simulink model "DSB_SC_coherent_2020b"  (R2020b)
settings: Solver=ode45  StartTime=0.0  StopTime=50  RelTol=1e-3  EnableMultiTasking=on
values from neighbouring files (symbols this model uses):
  seed = input('Enter your student ID: ')    [DSBAMsignals.m]    (also in DSBAMsignals_rand.m; DSB_SC_sinusoidals.m)
libraries: dsparch4 x2
settings Model: Creator=morelos_zaragoza  LastModifiedBy=14083
settings DataIOCC: LimitDataPoints=on  SaveFormat=Array  SignalLoggingSaveFormat=ModelDataLogs  ReturnWorkspaceOutputs=off
settings OptimizationCC: ExpressionDepthLimit=2147483647  InitFltsAndDblsToZero=on  LifeSpan=inf
settings DebuggingCC: SaveWithParameterizedLinksMsg=none  UnderspecifiedInitializationDetection=Classic  MergeDetectMultiDrivingBlocksExec=none  SignalResolutionControl=TryResolveAllWithWarning  SolverPrmCheckMsg=warning  MultiTaskDSMMsg=warning  MultiTaskCondExecSysMsg=none  FcnCallInpInsideContextMsg=warning  StateNameClashWarn=warning  SFUnexpectedBacktrackingDiag=warning  SFNoUnconditionalDefaultTransitionDiag=warning  SFExecutionAtInitializationDiag=none  ArithmeticOperatorsInVariantConditions=warning
settings HardwareCC: ProdBitPerPointer=32  ProdBitPerSizeT=32  ProdBitPerPtrDiffT=32  ProdLargestAtomicFloat=None  ProdIntDivRoundTo=Undefined  ProdEndianess=Unspecified  ProdWordSize=32  ProdHWDeviceType=32-bit Generic
settings ModelReferenceCC: PropagateSignalLabelsOutOfModel=off
settings SFSimCC: SimUseLocalCustomCode=off  CustomCodeUndefinedFunction=UseInterfaceOnly
settings RTWCC: RTWUseLocalCustomCode=off
settings CodeAppCC: StateflowObjectComments=on
settings GRTTargetCC: TargetFcnLib=ansi_tfl_tmw.mat  TargetLangStandard=C89/C90 (ANSI)  CombineOutputUpdateFcns=off  GRTInterface=on
settings ConfigComp: CovMetricSettings=dw  CovSaveCumulativeToWorkspaceVar=on  CovSaveSingleToWorkspaceVar=on  CovExternalEMLEnable=off

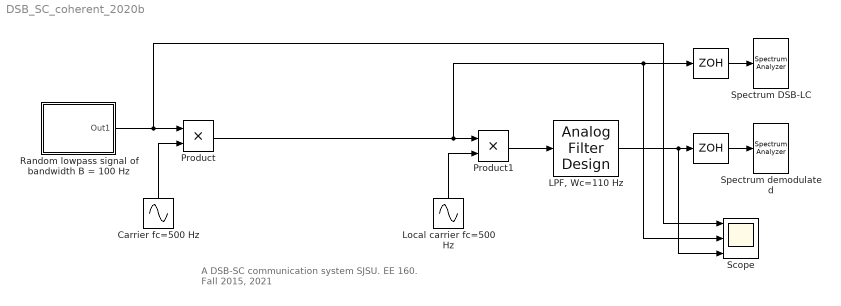
== system DSB_SC_coherent_2020b ==
  note: A DSB-SC communication system
      | SJSU. EE 160. Fall 2015, 2021
  "  " : ZeroOrderHold  SampleTime=1/(25*90)
  "   " : ZeroOrderHold  SampleTime=1/(25*90)
  "   Carrier fc=500 Hz" : Sin  Frequency=2*pi*500  SampleTime=0
  "LPF, Wc=110 Hz" : dsparch4/Analog Filter Design  method=Butterworth  filttype=Lowpass  N=2  Wlo=2*pi*110  Whi=2*pi*110  Rp=2  Rs=40
  Local carrier fc=500 Hz : Sin  Amplitude=2  Frequency=2*pi*500  SampleTime=0
  Product : Product  RndMeth=Zero
  Product1 : Product  RndMeth=Zero
  Random lowpass signal of bandwidth B = 100 Hz : Subsystem  TreatAsAtomicUnit=on
  Scope : Scope  NumInputPorts=3
  Spectrum DSB-LC : SpectrumAnalyzer
  Spectrum demodulated : SpectrumAnalyzer
  wires:
  Random lowpass signal of bandwidth B = 100 Hz/1(Out1) -> Product/1, Scope/1
  "   Carrier fc=500 Hz"/1 -> Product/2
  "  "/1 -> Spectrum DSB-LC/1
  "   "/1 -> Spectrum demodulated/1
  "LPF, Wc=110 Hz"/1 -> "   "/1, Scope/3
  Product/1 -> "  "/1, Scope/2, Product1/1
  Local carrier fc=500 Hz/1 -> Product1/2
  Product1/1 -> "LPF, Wc=110 Hz"/1

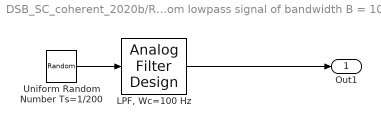
== system DSB_SC_coherent_2020b/Random lowpass signal of bandwidth B = 100 Hz ==
  "LPF, Wc=100 Hz" : dsparch4/Analog Filter Design  method=Butterworth  filttype=Lowpass  N=22  Wlo=2*pi*100  Whi=2*pi*110  Rp=2  Rs=40
  Uniform Random Number Ts=1/200 : UniformRandomNumber  Seed=seed  SampleTime=1/200
  Out1 : Outport
  wires:
  Uniform Random Number Ts=1/200/1 -> "LPF, Wc=100 Hz"/1
  "LPF, Wc=100 Hz"/1 -> Out1/1
